simulink model "PIDpointFollower"  (R2020b)
settings: Solver=VariableStepAuto  StartTime=0.0  StopTime=inf  RelTol=1e-3
PreLoadFcn:
  | ROSconfig
  | goalSignalSetup
PostLoadFcn:
  | RL_configParameters
InitFcn:
  | RL_configParameters
StartFcn:
  | gazeboSetup
StopFcn:
  | gazeboReset
  | goalreset
  | RL_loadResults
undefined symbols (not defined in the file): angmax, Angular, DiscIntNeverNeededParam, distThresh, Kd, Ki, Kp, Linear, vmax, wgain
libraries: simulink x4, robotlib x3, mobileRoboticsLib x1
PauseFcn:
  | gazeboPause
settings Model: Creator=Tyreeses'  LastModifiedBy=Tyreeses'

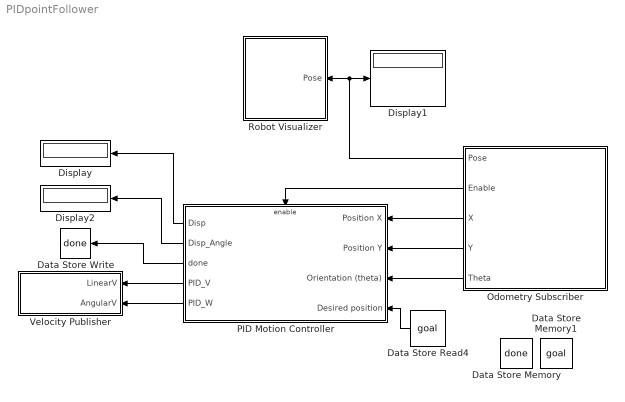
== system PIDpointFollower ==
  Data Store Memory : DataStoreMemory  DataStoreName=done  ReadBeforeWriteMsg=warning  WriteAfterWriteMsg=warning  WriteAfterReadMsg=warning  ShowAdditionalParam=off
  Data Store Memory1 : DataStoreMemory  DataStoreName=goal  ReadBeforeWriteMsg=warning  WriteAfterWriteMsg=warning  WriteAfterReadMsg=warning  InitialValue=goalpoint  VectorParams1D=off  ShowAdditionalParam=off
  Data Store Read4 : DataStoreRead  DataStoreName=goal  DataStoreElements=goal
  Data Store Write : DataStoreWrite  DataStoreName=done  DataStoreElements=done
  Display : Display
  Display1 : Display
  Display2 : Display
  Odometry Subscriber : Subsystem
  PID Motion Controller : Subsystem
  Robot Visualizer : Subsystem
  Velocity Publisher : Subsystem
  wires:
  PID Motion Controller/1(Disp) -> Display/1
  PID Motion Controller/2(Disp_Angle) -> Display2/1
  Data Store Read4/1 -> PID Motion Controller/4(Desired position)
  Odometry Subscriber/1(Pose) -> Robot Visualizer/1(Pose), Display1/1
  PID Motion Controller/5(PID_W) -> Velocity Publisher/2(AngularV)
  PID Motion Controller/4(PID_V) -> Velocity Publisher/1(LinearV)
  Odometry Subscriber/4(Y) -> PID Motion Controller/2(Position Y)
  Odometry Subscriber/3(X) -> PID Motion Controller/1(Position X)
  Odometry Subscriber/5(Theta) -> PID Motion Controller/3(Orientation (theta))
  Odometry Subscriber/2(Enable) -> PID Motion Controller/Enable
  PID Motion Controller/3(done) -> Data Store Write/1

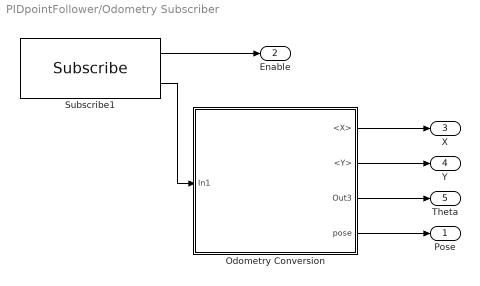
== system PIDpointFollower/Odometry Subscriber ==
  Odometry Conversion : Subsystem
  Subscribe1 : robotlib/Subscribe  topicSource=Select from ROS network  topic=/sim_p3at/odom  messageType=nav_msgs/Odometry  SampleTime=-1  legacyBusStruct=off  messageQueueLength=51
  Pose : Outport  VectorParamsAs1DForOutWhenUnconnected=off
  Enable : Outport  Port=2  VectorParamsAs1DForOutWhenUnconnected=off
  X : Outport  Port=3  VectorParamsAs1DForOutWhenUnconnected=off
  Y : Outport  Port=4  VectorParamsAs1DForOutWhenUnconnected=off
  Theta : Outport  Port=5  VectorParamsAs1DForOutWhenUnconnected=off
  wires:
  Subscribe1/1 -> Enable/1
  Subscribe1/2 -> Odometry Conversion/1(In1)
  Odometry Conversion/3(Out3) -> Theta/1
  Odometry Conversion/4(pose) -> Pose/1
  Odometry Conversion/1(<X>) -> X/1
  Odometry Conversion/2(<Y>) -> Y/1

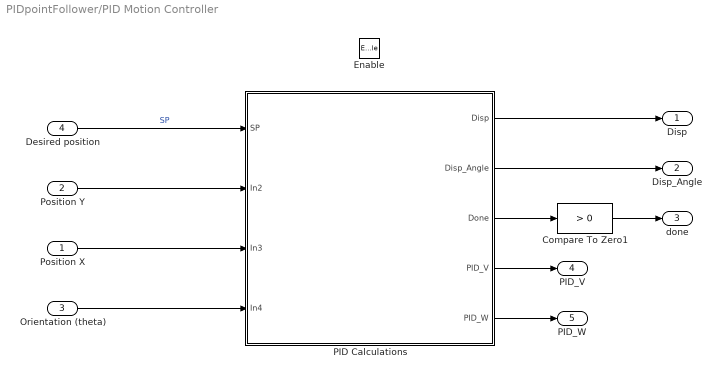
== system PIDpointFollower/PID Motion Controller ==
  Position X : Inport
  Position Y : Inport  Port=2
  Orientation (theta) : Inport  Port=3
  Desired position : Inport  Port=4
  Enable : EnablePort
  Compare To Zero1 : simulink/Logic and Bit Operations/Compare To Zero  relop=>  OutDataTypeStr=boolean
  PID Calculations : Subsystem
  Disp : Outport
  Disp_Angle : Outport  Port=2
  done : Outport  Port=3
  PID_V : Outport  Port=4
  PID_W : Outport  Port=5
  wires:
  Compare To Zero1/1 -> done/1
  PID Calculations/3(Done) -> Compare To Zero1/1
  Desired position/1 -> PID Calculations/1(SP)  "SP"
  Position Y/1 -> PID Calculations/2(In2)
  Position X/1 -> PID Calculations/3(In3)
  Orientation (theta)/1 -> PID Calculations/4(In4)
  PID Calculations/1(Disp) -> Disp/1
  PID Calculations/2(Disp_Angle) -> Disp_Angle/1
  PID Calculations/4(PID_V) -> PID_V/1
  PID Calculations/5(PID_W) -> PID_W/1

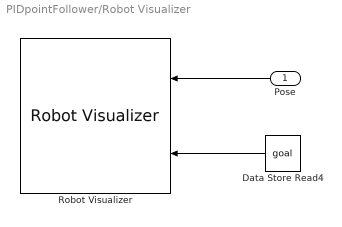
== system PIDpointFollower/Robot Visualizer ==
  Pose : Inport
  Data Store Read4 : DataStoreRead  DataStoreName=goal  DataStoreElements=goal
  Robot Visualizer : mobileRoboticsLib/Environments/Robot Visualizer  Priority=99  robotRadius=.34  showTrajectory=on  hasWaypoints=on  hasLidar=off  sensorOffset=[ 0 0 ]  scanAngles=0  hasObjDetector=off  objDetectorOffset=[ 0,0 ]  objDetectorAngle=0  objDetectorFOV=0  objDetectorMaxRange=0  objectColors=[1,0,0;0,1,0;0,0,1]  objectMarkers='s'
  wires:
  Pose/1 -> Robot Visualizer/1
  Data Store Read4/1 -> Robot Visualizer/2

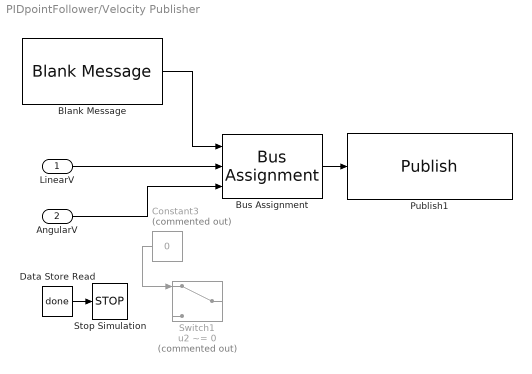
== system PIDpointFollower/Velocity Publisher ==
  LinearV : Inport
  AngularV : Inport  Port=2
  Blank Message : robotlib/Blank Message  messageClass=Message  entityType=geometry_msgs/Twist  messageType=geometry_msgs/Twist  SampleTime=-1  legacyBusStruct=off
  Bus Assignment : BusAssignment  DialogController=Simulink.DDGSource_BusAssignment  AssignedSignals=Linear.X,Angular.Z
  Constant3 : Constant  Commented=on  Value=0
  Data Store Read : DataStoreRead  DataStoreName=done
  Publish1 : robotlib/Publish  topicSource=Select from ROS network  topic=/sim_p3at/cmd_vel  messageType=geometry_msgs/Twist  legacyBusStruct=off  messageQueueLength=105
  Stop Simulation : Stop
  Switch1 : Switch  Commented=on  Criteria=u2 ~= 0
  wires:
  AngularV/1 -> Bus Assignment/3
  Bus Assignment/1 -> Publish1/1
  LinearV/1 -> Bus Assignment/2
  Blank Message/1 -> Bus Assignment/1
  Constant3/1 -> Switch1/1
  Data Store Read/1 -> Stop Simulation/1

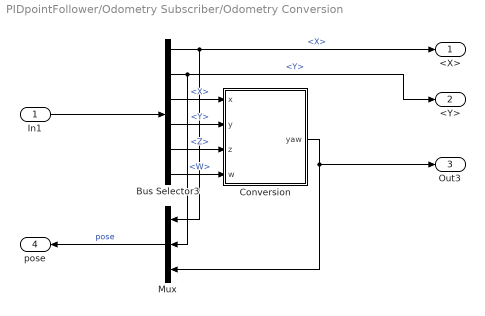
== system PIDpointFollower/Odometry Subscriber/Odometry Conversion ==
  In1 : Inport
  Bus Selector3 : BusSelector  OutputSignals=Pose.Pose.Position.X,Pose.Pose.Position.Y,Pose.Pose.Orientation.X,Pose.Pose.Orientation.Y,Pose.Pose.Orientation.Z,Pose.Pose.Orientation.W
  Conversion : MATLAB Function  TreatAsAtomicUnit=on
  Mux : Mux  Inputs=3
  <X> : Outport  VectorParamsAs1DForOutWhenUnconnected=off
  <Y> : Outport  Port=2  VectorParamsAs1DForOutWhenUnconnected=off
  Out3 : Outport  Port=3  VectorParamsAs1DForOutWhenUnconnected=off
  pose : Outport  Port=4  VectorParamsAs1DForOutWhenUnconnected=off
  wires:
  In1/1 -> Bus Selector3/1
  Bus Selector3/3 -> Conversion/1(x)  "<X>"
  Bus Selector3/4 -> Conversion/2(y)  "<Y>"
  Bus Selector3/5 -> Conversion/3(z)  "<Z>"
  Bus Selector3/6 -> Conversion/4(w)  "<W>"
  Conversion/1(yaw) -> Mux/3, Out3/1
  Bus Selector3/2 -> Mux/2, <Y>/1  "<Y>"
  Bus Selector3/1 -> Mux/1, <X>/1  "<X>"
  Mux/1 -> pose/1  "pose"

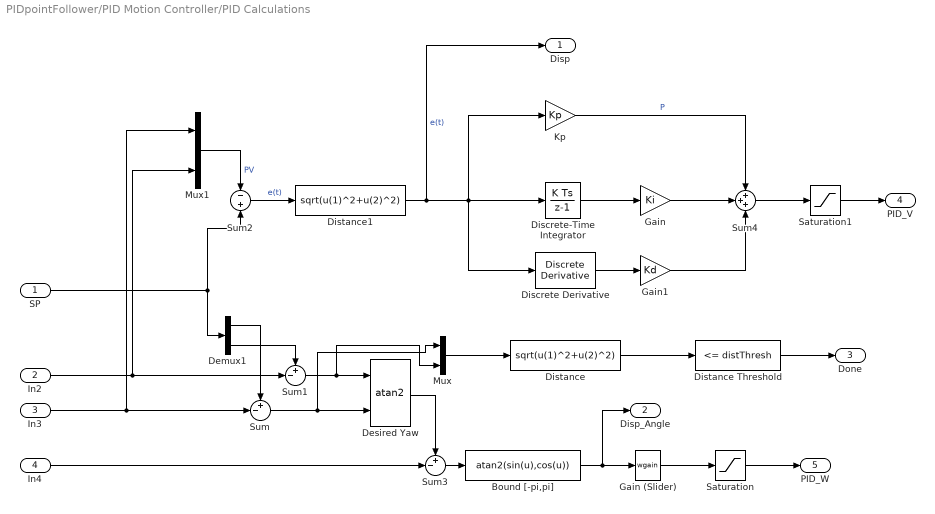
== system PIDpointFollower/PID Motion Controller/PID Calculations ==
  SP : Inport
  In2 : Inport  Port=2
  In3 : Inport  Port=3
  In4 : Inport  Port=4
  Bound [-pi,pi] : Fcn  Expr=atan2(sin(u),cos(u))
  Demux1 : Demux  Outputs=2
  Desired Yaw : Trigonometry  Operator=atan2
  Discrete Derivative : simulink/Discrete/Discrete Derivative  gainval=1  ICPrevScaledInput=0.0  OutMin=[]  OutMax=[]  OutDataType=fixdt(1, 16)  OutScaling=2^-10  DoSatur=off
  Discrete-Time Integrator : DiscreteIntegrator  gainval=1  SampleTime=-1  ICPrevOutput=DiscIntNeverNeededParam  ICPrevScaledInput=DiscIntNeverNeededParam
  Distance : Fcn  Expr=sqrt(u(1)^2+u(2)^2)
  Distance Threshold : simulink/Logic and Bit Operations/Compare To Constant  relop=<=  const=distThresh  OutDataTypeStr=boolean
  Distance1 : Fcn  Expr=sqrt(u(1)^2+u(2)^2)
  Gain : Gain  Gain=Ki
  Gain (Slider) : simulink/Math Operations/Slider Gain  gain=wgain  low=1  high=10
  Gain1 : Gain  Gain=Kd
  Kp : Gain  Gain=Kp
  Mux : Mux  Inputs=2
  Mux1 : Mux  Inputs=2
  Saturation : Saturate  UpperLimit=angmax  LowerLimit=-angmax
  Saturation1 : Saturate  UpperLimit=vmax  LowerLimit=-.5
  Sum : Sum  Inputs=+-|
  Sum1 : Sum  Inputs=+-|
  Sum2 : Sum  Inputs=-+
  Sum3 : Sum  Inputs=+-|
  Sum4 : Sum  Inputs=+++
  Disp : Outport
  Disp_Angle : Outport  Port=2
  Done : Outport  Port=3  VectorParamsAs1DForOutWhenUnconnected=off
  PID_V : Outport  Port=4  VectorParamsAs1DForOutWhenUnconnected=off
  PID_W : Outport  Port=5  VectorParamsAs1DForOutWhenUnconnected=off
  wires:
  In4/1 -> Sum3/2
  Desired Yaw/1 -> Sum3/1
  Sum/1 -> Desired Yaw/2, Mux/1
  Gain (Slider)/1 -> Saturation/1
  Saturation/1 -> PID_W/1
  Sum3/1 -> Bound [-pi,pi]/1
  Mux1/1 -> Sum2/1  "PV"
  Kp/1 -> Sum4/1  "P"
  Distance1/1 -> Disp/1, Kp/1, Discrete-Time Integrator/1, Discrete Derivative/1  "e(t)"
  Discrete-Time Integrator/1 -> Gain/1
  Demux1/1 -> Sum/1
  Demux1/2 -> Sum1/1
  Sum1/1 -> Desired Yaw/1, Mux/2
  SP/1 -> Demux1/1, Sum2/2
  In2/1 -> Sum1/2, Mux1/2
  In3/1 -> Sum/2, Mux1/1
  Distance/1 -> Distance Threshold/1
  Mux/1 -> Distance/1
  Bound [-pi,pi]/1 -> Disp_Angle/1, Gain (Slider)/1
  Sum2/1 -> Distance1/1  "e(t)"
  Gain/1 -> Sum4/2
  Sum4/1 -> Saturation1/1
  Discrete Derivative/1 -> Gain1/1
  Gain1/1 -> Sum4/3
  Distance Threshold/1 -> Done/1
  Saturation1/1 -> PID_V/1

== matlab function PIDpointFollower/Odometry Subscriber/Odometry Conversion/Conversion ==
  data: yaw output; x input; y input; z input; w input
function yaw  = quat2eul(x,y,z,w)
%#codegen

% Convert the quaternion to a yaw angle (zyx euler angle)
eul = quat2eul([w,x,y,z]);
yaw = eul(1);

end
